simulink model "Test2"  (R2019a)
settings: Solver=VariableStepAuto  StartTime=0.0  StopTime=t1+t2+t3+t4+t5+t6+t7  RelTol=1e-3
values from neighbouring files (symbols this model uses):
  A_continous_time = zeros(6,6)    [MPCDesigner_YAW.m]    (also in MPC_designer_X.m = zeros(10,10); MPC_designer_Z.m; NonTilting.m = zeros(10,10); RUN_simulation.m)
  A_dis_calc = expm(kSamplingTime*A_continous_time)    [MPC_designer_X.m]    (also in NonTilting.m; RUN_simulation.m; Simulacija_MPC_YAW_NELINEARNI.m; Simulacija_MPC_Z.m)
  B_continous_time = zeros(6,4)    [MPCDesigner_YAW.m]    (also in MPC_designer_X.m = zeros(10,4); MPC_designer_Z.m; NonTilting.m = zeros(10,4); RUN_simulation.m)
  B_dis_calc = integral_exp_A * B_continous_time    [MPC_designer_X.m]    (also in NonTilting.m; RUN_simulation.m; Simulacija_MPC_YAW_NELINEARNI.m; Simulacija_MPC_Z.m)
  kSamplingTime = 0.810    (= 0.81)    [MPCDesigner_YAW.m]    (also in MPC_designer_X.m = 0.1; MPC_designer_Z.m; NonTilting.m = 0.015; RUN_simulation.m = 0.015)
  t1 = 3.7182    [RUN_simulation.m]    (also in Simulacija_Roll.m = 1.64; ZaTest3.m = 18.591; ZaTest4.m = 18.591; proba_adam_simulink.m = 3.22580645161)
  t2 = 7.1656    [RUN_simulation.m]    (also in Simulacija_Roll.m = 1.8949; ZaTest3.m = 35.828; ZaTest4.m = 35.828; proba_adam_simulink.m = 2.41397650191)
  t3 = 3.7182    [RUN_simulation.m]    (also in Simulacija_Roll.m = 1.64; ZaTest3.m = 18.591; ZaTest4.m = 18.591; proba_adam_simulink.m = 3.22580645161)
  t4 = 0    [RUN_simulation.m]    (also in Simulacija_Roll.m; ZaTest3.m; ZaTest4.m; proba_adam_simulink.m)
  t5 = 3.7182    [RUN_simulation.m]    (also in Simulacija_Roll.m = 1.64; ZaTest3.m = 18.591; ZaTest4.m = 18.591; proba_adam_simulink.m = 3.22580645161)
  t6 = 7.1656    [RUN_simulation.m]    (also in Simulacija_Roll.m = 1.8949; ZaTest3.m = 35.828; ZaTest4.m = 35.828; proba_adam_simulink.m = 2.41397650191)
  theta_x = pomocni    [Preuredi.m]
libraries: simulink x5
settings Model: Creator=branko  LastModifiedBy=branko
settings DataIOCC: ReturnWorkspaceOutputs=off
settings DebuggingCC: ArithmeticOperatorsInVariantConditions=warning

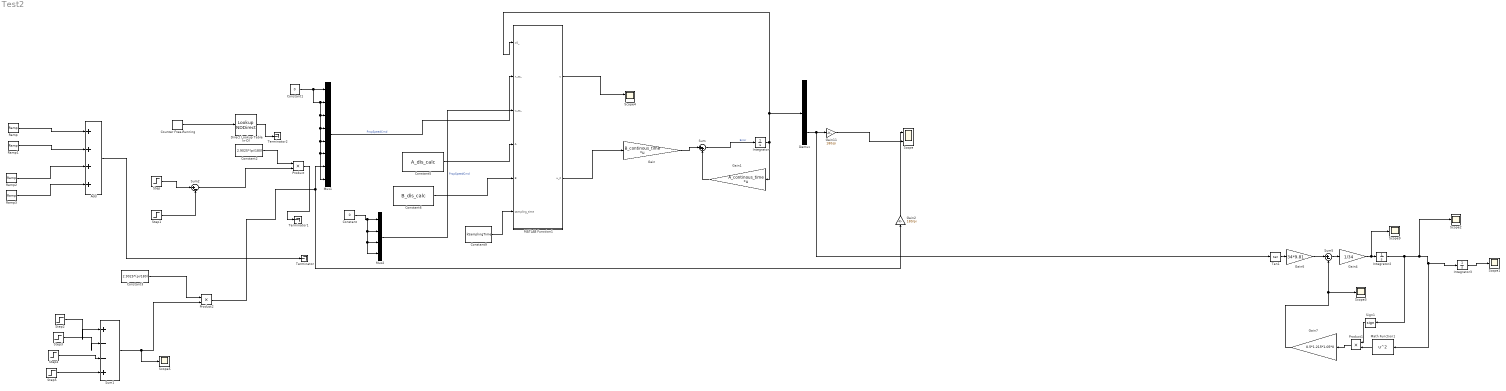
== system Test2 ==
  Add : Sum  Inputs=++++
  Constant : Constant  Value=0  OutDataTypeStr=double  SampleTime=-1
  Constant1 : Constant  Value=0  OutDataTypeStr=double  SampleTime=-1
  Constant2 : Constant  Value=2.9025*(pi/180)  OutDataTypeStr=double
  Constant3 : Constant  Value=2.9025*(pi/180)  OutDataTypeStr=double
  Constant5 : Constant  Value=A_dis_calc
  Constant6 : Constant  Value=B_dis_calc
  Constant9 : Constant  Value=kSamplingTime
  Counter Free-Running : simulink/Sources/Counter Free-Running  NumBits=32  tsamp=0.001
  Demux : Demux  Outputs=8
  Direct Lookup Table (n-D) : LookupNDDirect  NumberOfTableDimensions=1  Table=theta_x
  Gain : Gain  Gain=B_continous_time  Multiplication=Matrix(K*u)
  Gain1 : Gain  Gain=A_continous_time  Multiplication=Matrix(K*u)
  Gain11 : Gain  Gain=180/pi
  Gain2 : Gain  Gain=180/pi
  Gain4 : Gain  Gain=1/34
  Gain6 : Gain  Gain=34*9.81
  Gain7 : Gain  Gain=0.5*1.215*1.05*0
  Integrator : Integrator  InitialCondition=zeros(8,1)
  Integrator2 : Integrator
  Integrator3 : Integrator
  MATLAB Function1 : MATLAB Function  TreatAsAtomicUnit=on  SystemSampleTime=kSamplingTime
  Math Function1 : Math  Operator=square  SaturateOnIntegerOverflow=on
  Mux1 : Mux  Inputs=8
  Mux2 : Mux
  Product : Product
  Product1 : Product
  Product2 : Product
  Ramp : simulink/Sources/Ramp  slope=12*pi/180  start=0  InitialOutput=0
  Ramp1 : simulink/Sources/Ramp  slope=-12*pi/180  start=1.5  InitialOutput=0
  Ramp2 : simulink/Sources/Ramp  slope=-12*pi/180  start=3.0  InitialOutput=0
  Ramp3 : simulink/Sources/Ramp  slope=12*pi/180  start=4.5  InitialOutput=0
  Scope : Scope  NumInputPorts=2
  Scope{1..3,5,9} (5 alike) : Scope
  Scope4 : Scope  NumInputPorts=2
  Sign1 : Signum
  Step : Step  Time=0  SampleTime=0
  Step1 : Step  Time=5  SampleTime=0
  Step2 : Step  Time=0  SampleTime=0
  Step3 : Step  Time=t1+t2  SampleTime=0
  Step4 : Step  Time=t1+t2+t3+t4  SampleTime=0
  Step5 : Step  Time=t1+t2+t3+t4+t5+t6  SampleTime=0
  Sum : Sum  Inputs=|++
  Sum1 : Sum  Inputs=|+--+
  Sum2 : Sum  Inputs=|+-
  Sum5 : Sum  Inputs=|+-
  Tan1 : Trigonometry  Operator=tan
  Terminator : Terminator
  Terminator1 : Terminator
  Terminator2 : Terminator
  wires:
  Mux1/1 -> MATLAB Function1/2(x_ss_)  "PropSpeedCmd"
  Mux2/1 -> MATLAB Function1/3(u_ss_)  "PropSpeedCmd"
  Constant/1 -> Mux2/4, Mux2/3, Mux2/2, Mux2/1
  Constant1/1 -> Mux1/6, Mux1/8, Mux1/5, Mux1/4, Mux1/3, Mux1/2, Mux1/1
  Gain/1 -> Sum/1
  Gain1/1 -> Sum/2
  Sum/1 -> Integrator/1  "Error"
  Integrator/1 -> Gain1/1, MATLAB Function1/1(x0_), Demux/1
  Demux/7 -> Tan1/1, Gain11/1
  MATLAB Function1/1(u) -> Scope4/1
  Step/1 -> Sum2/1
  Constant2/1 -> Product/1
  Sum2/1 -> Product/2
  Step1/1 -> Sum2/2
  Constant5/1 -> MATLAB Function1/4(A)
  Constant6/1 -> MATLAB Function1/5(B)
  MATLAB Function1/2(u_2) -> Gain/1
  Product2/1 -> Mux1/7, Gain2/1
  Gain2/1 -> Scope/1
  Ramp/1 -> Add/1
  Ramp1/1 -> Add/2
  Ramp2/1 -> Add/3
  Ramp3/1 -> Add/4
  Add/1 -> Terminator/1
  Constant9/1 -> MATLAB Function1/6(sampling_time)
  Sum5/1 -> Gain4/1
  Product1/1 -> Gain7/1
  Gain4/1 -> Scope9/1, Integrator2/1
  Math Function1/1 -> Product1/2
  Sign1/1 -> Product1/1
  Gain7/1 -> Scope3/1, Sum5/2
  Gain6/1 -> Sum5/1
  Tan1/1 -> Gain6/1
  Gain11/1 -> Scope/2
  Integrator2/1 -> Sign1/1, Scope2/1, Math Function1/1, Integrator3/1
  Integrator3/1 -> Scope1/1
  Counter Free-Running/1 -> Direct Lookup Table (n-D)/1
  Sum1/1 -> Scope5/1, Product2/2
  Constant3/1 -> Product2/1
  Step2/1 -> Sum1/1
  Step4/1 -> Sum1/3
  Step5/1 -> Sum1/4
  Step3/1 -> Sum1/2
  Direct Lookup Table (n-D)/1 -> Terminator2/1
  Product/1 -> Terminator1/1

== matlab function Test2/MATLAB Function1 ==
  settings: updateMethod=DISCRETE
  data: x0_ input; u output; x_ss_ input; u_ss_ input; u_2 output; A input; B input; sampling_time input
function [u, u_2]  = adam(x0_, x_ss_, u_ss_, A, B, sampling_time)

persistent new_desire_state  pred_horizon control_horizon max_iter    R R_delta ...
           scale_MV_inv Q  scale_OV_inv gradients gradient_past ...
           gradient_square_past gradient_past_tilda gradient_square_past_tilda ...
           x_states deriv_wrt_u epsilon rho1 rho2 delta num_heuristic_vars ...
           u_past u_current lambdas_x lambdas_u lambdas_u_ref u_horizon ref_old t u_last_step ...
           du_max u_max index_first



       
if(isempty(new_desire_state) )
    index_first = 0;
    u_last_step = zeros(4, 1);
    du_max = zeros(4,2);
    u_max = zeros(4,2);
    
    du_max(1,1) = sampling_time* 2;
    du_max(1,2) = -sampling_time * 2;
    du_max(2,1) = sampling_time * 2;
    du_max(2,2) = -sampling_time * 2;
    du_max(3,1) = 1*(sampling_time/0.01);
    du_max(3,2) = -1*(sampling_time/0.01);
    du_max(4,1) = 1*(sampling_time/0.01);
    du_max(4,2) = -1*(sampling_time/0.01);
    
    u_max(1,1) = 0.6 / 2 - 0.01;
    u_max(1,2) = -u_max(1,1);
    u_max(2,1) = 0.6 / 2 - 0.01;
    u_max(2,2) = -u_max(1,1);
    u_max(3,1) = 50;
    u_max(3,2) = -50;
    u_max(4,1) = 50;
    u_max(4,2) = -50;
    
    ref_old  = x_ss_;
    t = 0.0;
    epsilon = 0.04;
	rho1 = 0.9;
	rho2 = 0.999;
	delta = 1e-7;
max_iter = 5;
control_horizon = 5;
pred_horizon = 14;
num_heuristic_vars = 2;
gradients = zeros(num_heuristic_vars*control_horizon,1 );
gradient_past = zeros(num_heuristic_vars*control_horizon,1 );
gradient_past_tilda = zeros(num_heuristic_vars*control_horizon,1 );
gradient_square_past_tilda = zeros(num_heuristic_vars*control_horizon,1 );
gradient_square_past = zeros(num_heuristic_vars*control_horizon,1 );
new_desire_state = true;
scale_OV_inv = inv(diag([0.58, 4.0, 0.58, 4.0, 800, 800, 0.5236, 0.5236]));

scale_MV_inv = inv(diag([0.58, 0.58, 100, 100]));



%old
R =diag([0.67670, 0.67670, 0.13534000, 0.13534000]);
R_delta = diag([0.738879858135067, 0.738879858135067, 0.007388798581351,0.007388798581351]);
Q = diag([ 0.135340000000000,0.002706800000000,  0.1353400, 0.002706800, 0.002706800, 0.002706800,9508.7068000, 9.676700]);

%new


% 
% A =[    0.4271,    0.0223,         0,         0,         0,         0,         0 ,        0;
%    -8.7243,   -0.1501,         0,         0,         0,         0,         0,         0;
%          0,         0,    0.4271,    0.0223,         0,         0,         0,         0;
%          0,         0,   -8.7243,   -0.1501,         0,         0,         0,         0;
%          0,         0,         0,         0,    0.7300,         0,         0,         0;
%          0,         0,         0,         0,         0,    0.7300,         0,         0;
%     0.0090,    0.0005,    0.0090,    0.0005,    0.0001,   -0.0001,    1.0000,    0.0787;
%     0.1699,    0.0113,    0.1699,    0.0113,    0.0028,   -0.0028,         0 ,   1.0000];
%     
% B =[ 0.5729,         0 ,        0 ,        0;
%     8.7243,         0   ,      0 ,        0;
%          0,    0.5729  ,       0 ,        0;
%          0,    8.7243 ,        0 ,        0;
%          0,         0 ,   0.2700 ,        0;
%          0,         0 ,        0 ,   0.2700;
%    -0.0037,   -0.0037,    0.0000 ,  -0.0000;
%    -0.0347,   -0.0347,    0.0005 ,  -0.0005];



x_states = zeros(size(A, 1), pred_horizon+1);
deriv_wrt_u =  zeros(size(B,2), control_horizon);
u_past = zeros(size(B,2), 1);
u_current = zeros(size(B,2), 1);
u_ss_ = zeros(size(B,2), 1);
lambdas_x = zeros(size(A, 1), pred_horizon);
lambdas_u = zeros(size(B,2), pred_horizon);
u_horizon = zeros(size(B,2), pred_horizon);
lambdas_u_ref = zeros(size(B,2), pred_horizon);

end




residuum_signal =0.0;
residuum_state =0.0;

u = zeros(size(B,2), 1);

x = zeros(control_horizon *num_heuristic_vars,1);
change_x = zeros(control_horizon *num_heuristic_vars,1);

if(sum(x_ss_ - ref_old, 'double') < 1e-6)
   new_desire_state = false; 
else
    new_desire_state = true;

end

for iter = 1:max_iter
x_states(:,1) = x0_ ;
deriv_wrt_u = 0*deriv_wrt_u;
u_past = zeros(size(B,2), 1);% u_current*1;

if (new_desire_state) 
		new_desire_state = false;
		gradient_past = 0*gradient_past;
		gradient_square_past = 0*gradient_square_past;
		t = 0.0;
end

for i = 1:pred_horizon
    if(i <= control_horizon)
        u(1,1) = x(0*control_horizon  + i);
        u(2,1) = x(0*control_horizon  + i);
        u(3,1) = x(1*control_horizon  + i);
        u(4,1) = -x(1*control_horizon  + i);
    end
    
    
    
    x_states(:,i+1) = A * x_states(:,i) + B * u; 
    lambdas_x(:,i) = -1*x_ss_ + x_states(:,i+1); 
    lambdas_u(:,i) = u - u_past; 
    lambdas_u_ref(:, i) = u - u_ss_; 
 
    %derivation of u
    if(i <= control_horizon)
        deriv_wrt_u(:, i) = (2*R*u) -2*R*u_ss_  + (4*R_delta*u) -2*R_delta*u_past + deriv_wrt_u(:, i) ;
        
        if(i > 1)
            deriv_wrt_u(:, i-1) = deriv_wrt_u(:, i-1) -2*R_delta*u ;
        end
    else
        deriv_wrt_u(:, control_horizon) = deriv_wrt_u(:, control_horizon) + (2*R*u) -2*R*u_ss_  + (4*R_delta*u)+ (-2*R_delta*u_past) ;
        deriv_wrt_u(:, control_horizon) = deriv_wrt_u(:, control_horizon) -2*R_delta*u ;
    end
    
    %derivation of x
    for j = 1:i
        if(j <= control_horizon && i <= control_horizon)
            
            deriv_wrt_u(:,j) = deriv_wrt_u(:,j) + transpose(transpose( 2*Q*x_states(:,i+1) - 2*Q*x_ss_ )*(A^(i-j))*B); 
        else
            if(j > control_horizon)
                deriv_wrt_u(:,control_horizon) =deriv_wrt_u(:,control_horizon) +  transpose(transpose((2*Q*x_states(:,i+1) - 2*Q*x_ss_))*(A^(i-j))*B); 
            else
                deriv_wrt_u(:,j) =deriv_wrt_u(:,j) + transpose(transpose( 2*Q*x_states(:,i+1) - 2*Q*x_ss_ )*(A^(i-j))*B); 
            end
        end
    end
    u_past = u;
end


lambdas_u_ref =scale_MV_inv * lambdas_u_ref;
lambdas_u = scale_MV_inv * lambdas_u;
lambdas_x = scale_OV_inv * lambdas_x;
residuum_signal=sum((lambdas_u_ref.*(R*lambdas_u_ref)),'double')  + sum((lambdas_u.*(R_delta*lambdas_u)),'double'); 
residuum_state=sum((lambdas_x.*(Q*lambdas_x)),'double') ; 
        
residuum =  residuum_signal +  residuum_state;

for iter_der = 1:control_horizon
    gradients(iter_der, 1) = 2 * deriv_wrt_u(1, iter_der);
    gradients(iter_der + control_horizon, 1) = 2 * deriv_wrt_u(3, iter_der);
end

gradient_square_past = (rho2*gradient_square_past + (1 - rho2)*gradients.*(gradients));

gradient_past = (rho1*gradient_past + (1 - rho1)*gradients);

t  = t +1.0;

for adam_iter = 1:control_horizon *num_heuristic_vars
    gradient_past_tilda(adam_iter, 1) = (gradient_past(adam_iter, 1)) / (1.0 - (rho1^t));
	gradient_square_past_tilda(adam_iter, 1) = (gradient_square_past(adam_iter, 1)) / (1.0 - (rho2^t));
		

end

for adam_iter = 1:control_horizon *num_heuristic_vars
    change_x(adam_iter, 1) = -1 * (epsilon * gradient_past_tilda(adam_iter, 1)) / (sqrt(gradient_square_past_tilda(adam_iter, 1)) + delta);

end

x = (x + change_x);
end

u(1,1) = x(0*control_horizon  + 1);
u(2,1) = x(0*control_horizon  + 1);
u(3,1) = x(1*control_horizon  + 1);
u(4,1) = -x(1*control_horizon  + 1);

u_2 = u;
for iter_m = 1:4
    if(u_2(iter_m,1) > ( u_last_step(iter_m,1)+du_max(iter_m,1) ))
        u_2(iter_m,1) =  u_last_step(iter_m,1)+du_max(iter_m,1);
    elseif (u_2(iter_m,1) < ( u_last_step(iter_m,1)+du_max(iter_m,2) ))
        u_2(iter_m,1) =  u_last_step(iter_m,1)+du_max(iter_m,2);
    end
    
    if(u_2(iter_m,1) > u_max(iter_m,1) )
        u_2(iter_m,1) =  u_max(iter_m,1);
    elseif(u_2(iter_m,1) < u_max(iter_m,2))
        u_2(iter_m,1) =  u_max(iter_m,2);
    end
    
    
end

u_last_step = u_2;
end
